simulink model "I_SeatHeatingController__imple"  (R2017b)
settings: Solver=FixedStepDiscrete  StartTime=0.0  StopTime=10.0  FixedStep=1  RelTol=1e-3
PreLoadFcn:
  | sl_refresh_customizations
  | bus_Simulink
model workspace (MAT data in the model file):
  ESD_URL = 'http://127.0.0.1:63320/node?ref=r%3A4478b7d6-4519-4ad9-8c44-5a24e1aa32dc%28SeatHeater%29%2F3983288832293147565'
settings Model: Creator=eh6qym  LastModifiedBy=eh6qym
settings OptimizationCC: DefaultParameterBehavior=Inlined  PassReuseOutputArgsAs=Individual arguments  ZeroExternalMemoryAtStartup=off
settings DebuggingCC: SignalRangeChecking=error  InheritedTsInSrcMsg=none  ParameterTunabilityLossMsg=error
settings SFSimCC: MATLABDynamicMemAlloc=off
settings RTWCC: SystemTargetFile=esd_ert.tlc  GenCodeOnly=on  TemplateMakefile=ert_default_tmf  Description=ESD  GenerateReport=on  IncludeHyperlinkInReport=on  LaunchReport=on  GenerateTraceInfo=on  GenerateTraceReport=on  GenerateTraceReportSl=on  GenerateTraceReportSf=on  GenerateTraceReportEml=on
settings CodeAppCC: ForceParamTrailComments=on  IgnoreCustomStorageClasses=off  OperatorAnnotations=on  SimulinkDataObjDesc=on  SFDataObjDesc=on  InsertBlockDesc=on
settings STFCustomTargetCC: TargetLangStandard=C99 (ISO)  MultiwordLength=256  GenerateSampleERTMain=on  IncludeMdlTerminateFcn=off  CombineOutputUpdateFcns=on  CombineSignalStateStructs=on  SuppressErrorStatus=on  ERTCustomFileBanners=on  MultiInstanceERTCode=on  CodeInterfacePackaging=Reusable function  SupportContinuousTime=off  SupportNonInlinedSFcns=off  RemoveDisableFunc=on  RemoveResetFunc=on  MATLABClassNameForMDSCustomization=Simulink.SoftwareTarget.ERTCustomization  GRTInterface=off  SystemTargetFile=esd_ert.tlc
settings ERTTargetCC: TargetLangStandard=C99 (ISO)  GenerateSampleERTMain=on  ParMdlRefBuildCompliant=off  CompOptLevelCompliant=off  ConcurrentExecutionCompliant=off  IncludeMdlTerminateFcn=off  CombineSignalStateStructs=on  SuppressErrorStatus=on  MultiInstanceERTCode=on  CodeInterfacePackaging=Reusable function  RemoveDisableFunc=on  ModelStepFunctionPrototypeControlCompliant=off  CPPClassGenCompliant=off  UseToolchainInfoCompliant=off  InlinedParameterPlacement=NonHierarchical  ERTCustomFileTemplate=example_file_process.tlc

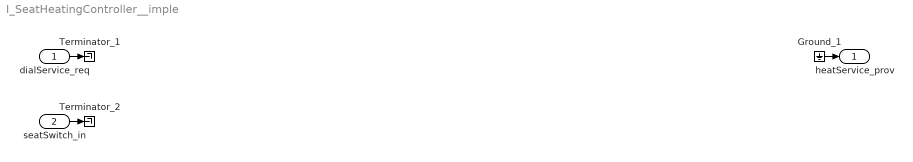
== system I_SeatHeatingController__imple ==
  dialService_req : Inport  OutDataTypeStr=Enum: IDialService_prov_t
  seatSwitch_in : Inport  Port=2  OutDataTypeStr=Bus: SeatSwitch_in_t  BusOutputAsStruct=on
  Ground_1 : Ground
  Terminator_1 : Terminator
  Terminator_2 : Terminator
  heatService_prov : Outport  OutDataTypeStr=Enum: IHeatService_prov_t
  wires:
  dialService_req/1 -> Terminator_1/1
  seatSwitch_in/1 -> Terminator_2/1
  Ground_1/1 -> heatService_prov/1
